simulink model "chap8_1sim"  (Simulink 7.7)
settings: Solver=ode45  SolverMode=SingleTasking  StartTime=0.0  StopTime=150  FixedStep=0.001  RelTol=1e-3
settings Model: Creator=ljk  LastModifiedBy=ljk  ExtModeTrigMode=oneshot  ExtModeArmWhenConnect=off
settings DataIOCC: LimitDataPoints=off  SignalLoggingName=sigsOut
settings OptimizationCC: BooleanDataType=off
settings DebuggingCC: SaveWithParameterizedLinksMsg=none  SignalResolutionControl=TryResolveAllWithWarning  SolverPrmCheckMsg=none  MultiTaskDSMMsg=warning  MultiTaskCondExecSysMsg=none  StrictBusMsg=None
settings HardwareCC: TargetUnknown=on
settings RTWCC: IncludeERTFirstTime=on

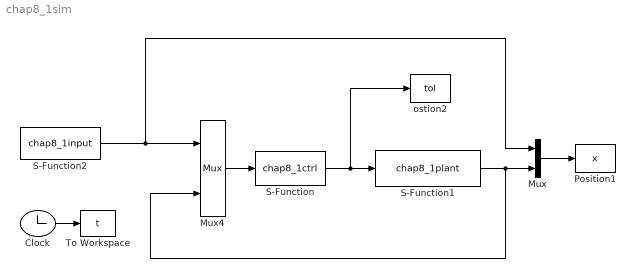
== system chap8_1sim ==
  Clock : Clock
  Mux : Mux  Inputs=2
  Mux4 : Mux  Inputs=2
  Position1 : ToWorkspace  VariableName=x  SampleTime=-1  SaveFormat=Array
  S-Function : S-Function  FunctionName=chap8_1ctrl  EnableBusSupport=off
  S-Function1 : S-Function  FunctionName=chap8_1plant  EnableBusSupport=off
  S-Function2 : S-Function  FunctionName=chap8_1input  EnableBusSupport=off
  To Workspace : ToWorkspace  VariableName=t  SampleTime=-1  SaveFormat=Array
  ostion2 : ToWorkspace  VariableName=tol  SampleTime=-1  SaveFormat=Array
  wires:
  Mux4/1 -> S-Function/1
  Clock/1 -> To Workspace/1
  S-Function2/1 -> Mux4/1, Mux/1
  S-Function/1 -> S-Function1/1, ostion2/1
  Mux/1 -> Position1/1
  S-Function1/1 -> Mux4/2, Mux/2
